simulink model "ButtonControlApp_Server"  (R2023a)
settings: Solver=FixedStepAuto  StartTime=0.0  StopTime=10.0  RelTol=1e-3
undefined symbols (not defined in the file): Back, Data_Display, Forward, Left, Right, SendData, Stop
libraries: androiduilib x6, androidcommunicationlib x1
settings Model: Creator=aqeel  LastModifiedBy=aqeel
settings OptimizationCC: EnhancedBackFolding=on  PassReuseOutputArgsAs=Individual arguments  ZeroExternalMemoryAtStartup=off  ZeroInternalMemoryAtStartup=off  MaxStackSize=64  OptimizeBlockOrder=speed  DifferentSizesBufferReuse=on  OptimizationCustomize=off  EfficientTunableParamExpr=on
settings DebuggingCC: ParameterTunabilityLossMsg=error
settings HardwareCC: ProdBitPerPointer=32  ProdBitPerSizeT=32  ProdBitPerPtrDiffT=32  ProdLargestAtomicInteger=Long  ProdLargestAtomicFloat=Double  ProdWordSize=32  ProdHWDeviceType=ARM Compatible->ARM Cortex
settings SFSimCC: MATLABDynamicMemAlloc=off
settings RTWCC: Description=Embedded Coder  SystemTargetFile=ert.tlc  HardwareBoard=Android Device  TLCOptions="-aInlineSetEventsForThisBaseRateFcn=TLC_FALSE -aSuppressMultiTaskScheduler=TLC_FALSE  -aRateBasedStepFcn=0"  TemplateMakefile=ert_default_tmf  RTWVerbose=off  Toolchain=Android SDK/NDK Tools
settings CodeAppCC: ForceParamTrailComments=on  IgnoreCustomStorageClasses=off  OperatorAnnotations=on  SimulinkDataObjDesc=on  SFDataObjDesc=on  InsertBlockDesc=on

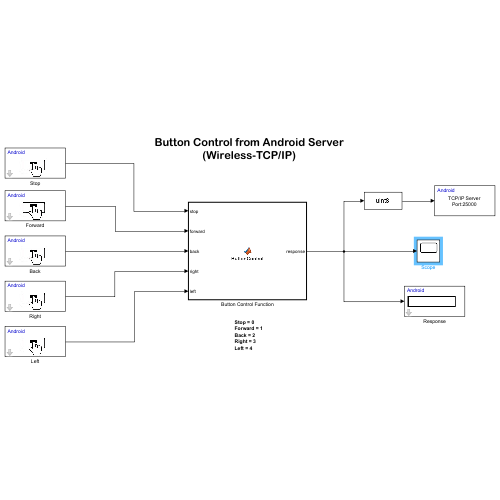
[thumbnail: Simulink's stored preview of the top-level diagram]
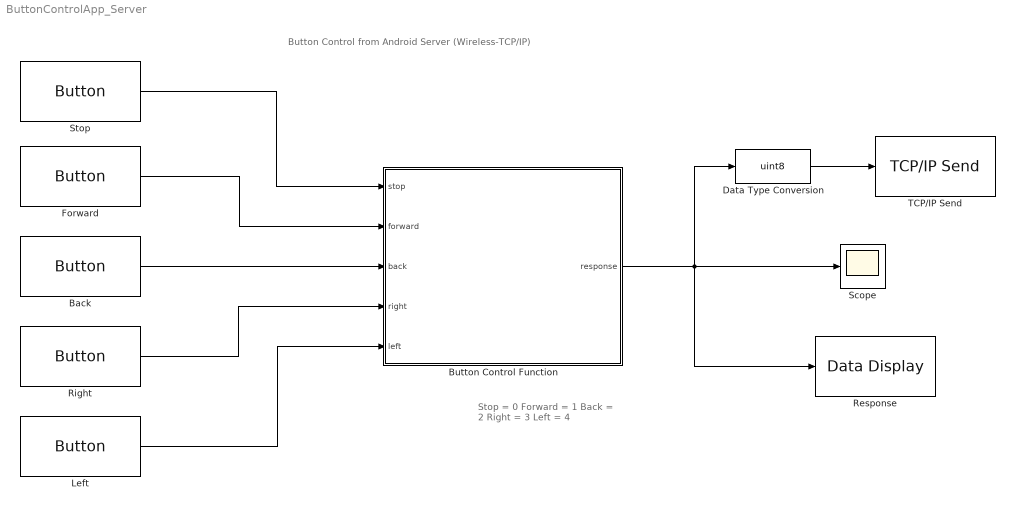
== system ButtonControlApp_Server ==
  note: Button Control from Android Server (Wireless-TCP/IP)
  note: Stop = 0
      | Forward = 1
      | Back = 2
      | Right = 3
      | Left = 4
  Back : androiduilib/Button  ButtonState=Not pressed  ButtonId=SendData/Back  State=off  SampleTime=0.1  BlockPlatform=Android
  Button Control Function : MATLAB Function  TreatAsAtomicUnit=on
  Data Type Conversion : DataTypeConversion  OutDataTypeStr=uint8  SaturateOnIntegerOverflow=off  RndMeth=Floor
  Forward : androiduilib/Button  ButtonState=Not pressed  ButtonId=SendData/Forward  State=off  SampleTime=0.1  BlockPlatform=Android
  Left : androiduilib/Button  ButtonState=Not pressed  ButtonId=SendData/Left  State=off  SampleTime=0.1  BlockPlatform=Android
  Response : androiduilib/Data Display  DataDisplayId=SendData/Data_Display  Format=Float  Precision=6  SimulateUsing=Code generation  blockPlatform=Android
  Right : androiduilib/Button  ButtonState=Not pressed  ButtonId=SendData/Right  State=off  SampleTime=0.1  BlockPlatform=Android
  Scope : Scope
  Stop : androiduilib/Button  ButtonState=Not pressed  ButtonId=SendData/Stop  State=off  SampleTime=0.1  BlockPlatform=Android
  TCP/IP Send : androidcommunicationlib/TCP//IP Send  TCPSendId=SendData/TCP//IP_Send  Mode_=Server  LocalServerPort_=25000  RemoteAddr_=105.225.146.89  RemoteServerPort_=25000  ClientPortBindingSelection_=off  ClientPortToBind_=35000  BlockingMode_=off  BlockTimeout_=0.1
  wires:
  Stop/1 -> Button Control Function/1(stop)
  Forward/1 -> Button Control Function/2(forward)
  Back/1 -> Button Control Function/3(back)
  Right/1 -> Button Control Function/4(right)
  Left/1 -> Button Control Function/5(left)
  Button Control Function/1(response) -> Response/1, Scope/1, Data Type Conversion/1
  Data Type Conversion/1 -> TCP/IP Send/1

== matlab function ButtonControlApp_Server/Button Control Function ==
  data: stop input; response output; forward input; back input; right input; left input
%Function to control Arduino robot using the android device via serial usb.
%Robot Controls:
%response = 0 --> Stop
%response = 1 --> Forward
%response = 2 --> Reverse
%response = 3 --> Right
%response = 4 --> Left

function response = ButtonControl(stop,forward,back,right,left)
Buttons=[stop,forward,back,right,left];
if sum(Buttons)==1
    if stop == 1
        response = 0;
    elseif forward==1
        response =1;
    elseif back ==1
        response=2;
    elseif right ==1
        response=3;
    elseif left==1
        response=4;
    else
        response=0;
    end
else
    response=0;
end
